simulink model "VDCHyd2022a"  (R2022a)
settings: Solver=daessc  StartTime=0.0  StopTime=simulationEndTime  FixedStep=0.001  RelTol=1e-2
values from neighbouring files (symbols this model uses):
  aux = thetaXrLB(i)    [initInertiaUpdate.m]
  Bc1_V = [0;0;0;0;0;0]    [InitializeSimulationParameters.m]
  Bc1_Vr = [0;0;0;0;0;0]    [InitializeSimulationParameters.m]
  D22Fr = [0;0;0;0;0;0]    [InitializeSimulationParameters.m]
  filtDF = init2ndOrderLowPassFilter(filtDF.cutOffFrequency,1,controller.dT)    [initializeLowPassFilters.m]
  filtDV = init2ndOrderLowPassFilter(filtDV.cutOffFrequency,1,controller.dT)    [initializeLowPassFilters.m]
  filtEnc = init2ndOrderLowPassFilter(filtEnc.cutOffFrequency,1,controller.dT)    [initializeLowPassFilters.m]
  filtPres = init2ndOrderLowPassFilter(filtPres.cutOffFrequency,1,controller.dT)    [initializeLowPassFilters.m]
  MODE = 1    [RUN_ME.m]
  s = tf('s')    [init2ndOrderLowPassFilter.m]
undefined symbols (not defined in the file or in its folder): B11_r_B11Tc1, B11_V, B11_Vr, B11Ftot_r, B12_r_B12Tc2, B12_Rot_Tc2, B12_U_Tc2, B12_V, B12_Vr, B12Ftot_r, B31_r_B31B41, B31_V, B31_Vr, B31FTot_r, B32_r_B32B42, B32_Rot_B42, B32_U_B42, B32_V, B32_Vr, B32FTot_r, B41_r_B41Tc1, B41_V, B41_Vr, B41FTot_r, B42_r_B42Tc2, B42_Rot_Tc2, B42_U_Tc2, B42_V, B42_Vr, B42FTot_r, B52_r_B52P32, B52_Rot_P32, B52_U_P32, B52_V, B52_Vr, B52Ftot_r, Bc1_r_Bc1B11, Bc1_r_Bc1B31, Bc1FTot_r, Bc2_r_Bc2B12, Bc2_r_Bc2B32, Bc2_Rot_B12, Bc2_Rot_B32, Bc2_U_B12, Bc2_U_B32, Bc2_V, Bc2_Vr, Bc2Tot_r, controller, cyl1, cyl2, cylT2, D22_V, D22_Vr, DiscIntNeverNeededParam, dq1, dq11, dq11r, dq12, dq12r ... (+119)
libraries: sm_lib x34, nesl_utility x15, simulink x11, dspinverses x1
(part 4 of 12)

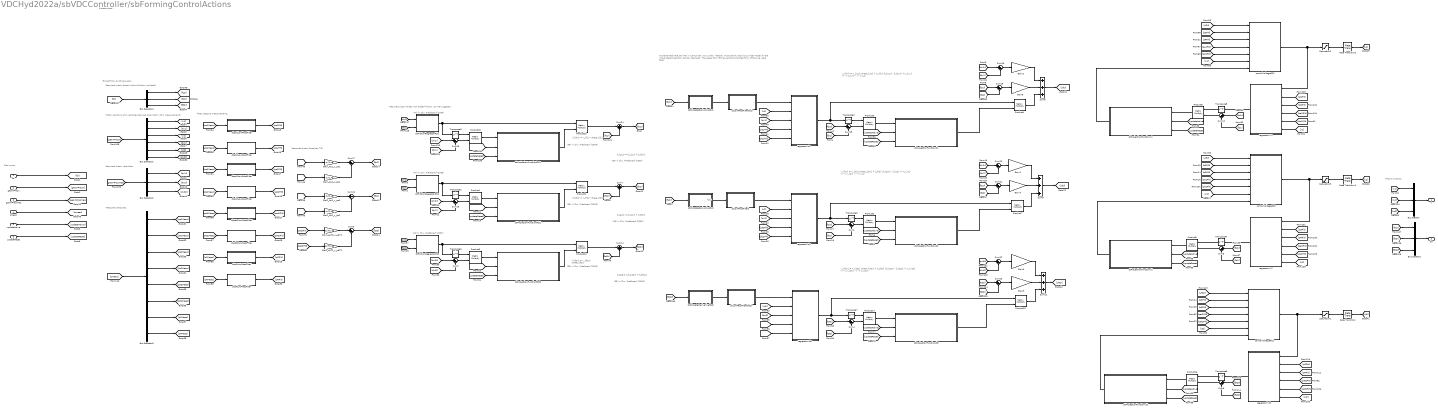
== system VDCHyd2022a/sbVDCController/sbFormingControlActions ==
  note: u_{f1r} = Y_{d1} \theta_{d1} + k_{f1} (f_{p1r} - f_{p1}) + k_{x1} (x^{'}_{1r} - x^{'}_1)
  note: fp2r
  note: Extract from existing buses...
  note: Get inputs...
  note: Pass to outputs...
  note: Process data...
  note: Filter pressure measurements.
  note: Measured piston force per (79).
  note: Required piston forces with added friction, as (78) suggests.
  note: Implemented here per (43) in (Lampinen, Koivumäki, Mattila): Improved Hydraulic Cylinder Model for the Virtual Decomposition Control Approach. The paper form (90) gives the simplified form of the one used here.
  note: Required piston forces (without friction included).
  note: Piston positions and velocities derived analytically from measurements.
  note: Required piston velocities.
  note: Measured pressures.
  note: f_{f1r} = Y_{f1}* \theta_{f1}
  note: f_{p1r} = f_{c1r} + f_{f1r}
  note: f_{f2r} = Y_{f2}* \theta_{f2}
  note: f_{p2r} = f_{c2r} + f_{f2r}
  note: f_{ft2r} = Y_{ft2}* \theta_{ft2}
  note: f_{pt2r} = f_{ct2r} + f_{ft2r}
  note: (40) in Zhu, Piedboeuf (2005)
  note: (40) in Zhu, Piedboeuf (2005)
  note: (40) in Zhu, Piedboeuf (2005)
  note: (39) in Zhu, Piedboeuf (2005)
  note: (39) in Zhu, Piedboeuf (2005)
  note: (39) in Zhu, Piedboeuf (2005)
  note: (38) in Zhu, Piedboeuf (2005)
  note: (38) in Zhu, Piedboeuf (2005)
  note: (38) in Zhu, Piedboeuf (2005)
  note: u_{f2r} = Y_{d2} \theta_{d2} + k_{f2} (f_{p2r} - f_{p2}) + k_{x2} (x^{'}_{2r} - x^{'}_2)
  note: u_{ft2r} = Y_{dt2} \theta_{dt2} + k_{ft2} (f_{pt2r} - f_{pt2}) + k_{xt2} (x^{'}_{t2r} - x^{'}_{t2})
  fcr : Inport
  geomPropX : Inport  Port=2
  geomPropXreq : Inport  Port=3
  pMeas : Inport  Port=4
  updateActive : Inport  Port=5
  updateReset : Inport  Port=6
  Bus Creator : BusCreator  Inputs=u1,u2,ut2
  Bus Creator1 : BusCreator  Inputs=fp1r,fp2r,fpt2r
  Bus Selector1 : BusSelector  OutputSignals=geomPropRS1.x1,geomPropRS1.dx1,geomPropRS2.x2,geomPropRS2.dx2,geomPropPS2.xt2,geomPropPS2.dxt2
  Bus Selector2 : BusSelector  OutputSignals=geomPropRS1req.dx1r,geomPropRS2req.dx2r,dxt2r
  Bus Selector3 : BusSelector  OutputSignals=pa1Measured,pb1Measured,pa2Measured,pb2Measured,pat2Measured,pbt2Measured,pSMeasured,pRMeasured
  Bus Selector4 : BusSelector  OutputSignals=fc1r,fc2r,fct2r
  Gain1 : Gain  Gain=controller.kx2
  Gain2 : Gain  Gain=controller.kx1
  Gain3 : Gain  Gain=controller.kxt2
  Gain4 : Gain  Gain=controller.kf2
  Gain8 : Gain  Gain=controller.kf1
  Gain9 : Gain  Gain=controller.kft2
  Gain_Aa1_x_pa1 : Gain  Gain=cyl1.Aa
  Gain_Aa2_x_pa2 : Gain  Gain=cyl2.Aa
  Gain_AaT2_x_paT2 : Gain  Gain=cylT2.Aa
  Gain_Ab1_x_pb1 : Gain  Gain=cyl1.Ab
  Gain_Ab2_x_pb2 : Gain  Gain=cyl2.Ab
  Gain_AbT2_x_pbT2 : Gain  Gain=cylT2.Ab
  Product{1..10,14..16,18,20} (15 alike) : Product  Multiplication=Matrix(*)
  Rate Transition : RateTransition  OutPortSampleTime=controller.dT
  Rate Transition1 : RateTransition  OutPortSampleTime=controller.dT
  Rate Transition2 : RateTransition  OutPortSampleTime=controller.dT
  Saturation1 : Saturate  UpperLimit=controller.ut2UppLim  LowerLimit=controller.ut2LowLim
  Saturation2 : Saturate  UpperLimit=controller.u1UppLim  LowerLimit=controller.u1LowLim
  Saturation3 : Saturate  UpperLimit=controller.u2UppLim  LowerLimit=controller.u2LowLim
  Sum{1..5,8,10,12..13,15..18,20..23,25} (18 alike) : Sum  Inputs=|+-
  Sum11 : Sum  Inputs=+++
  Sum14 : Sum  Inputs=|++
  Sum24 : Sum  Inputs=|++
  Sum6 : Sum  Inputs=+++
  Sum7 : Sum  Inputs=|++
  Sum9 : Sum  Inputs=+++
  Transpose{1..9} (9 alike) : Math  Operator=transpose
  controlVoltagePS2 : MATLAB Function  TreatAsAtomicUnit=on
  controlVoltageRS1 : MATLAB Function  TreatAsAtomicUnit=on
  controlVoltageRS2 : MATLAB Function  TreatAsAtomicUnit=on
  regressorYd1 : MATLAB Function  TreatAsAtomicUnit=on
  regressorYd2 : MATLAB Function  TreatAsAtomicUnit=on
  regressorYdt2 : MATLAB Function  TreatAsAtomicUnit=on
  regressorYv1 : MATLAB Function  TreatAsAtomicUnit=on
  regressorYv2 : MATLAB Function  TreatAsAtomicUnit=on
  regressorYvt2 : MATLAB Function  TreatAsAtomicUnit=on
  sbDiscreteDerivativefp1r : Subsystem
  sbDiscreteDerivativefp2r : Subsystem
  sbDiscreteDerivativefpt2r : Subsystem
  sbFrictionRegressorPS2 : Subsystem
  sbFrictionRegressorRS1 : Subsystem
  sbFrictionRegressorRS2 : Subsystem
  sbLowPassFilter2 : Subsystem
  sbLowPassFilterdfp1r : Subsystem
  sbLowPassFilterdfpt2r : Subsystem
  sbProjectionFunctiond1 : Subsystem
  sbProjectionFunctiond2 : Subsystem
  sbProjectionFunctiondt2 : Subsystem
  sbProjectionFunctionfRS1 : Subsystem
  sbProjectionFunctionfRS2 : Subsystem
  sbProjectionFunctionfRS3 : Subsystem
  sbProjectionFunctionv1 : Subsystem
  sbProjectionFunctionv2 : Subsystem
  sbProjectionFunctionvt2 : Subsystem
  sbpRLowPassFilter : Subsystem
  sbpSLowPassFilter : Subsystem
  sbpa1LowPassFilter : Subsystem
  sbpa2LowPassFilter : Subsystem
  sbpat2LowPassFilter : Subsystem
  sbpb1LowPassFilter : Subsystem
  sbpb2LowPassFilter : Subsystem
  sbpbt2LowPassFilter : Subsystem
  u : Outport
  fpr : Outport  Port=2
  wires:
  [uf1r] -> controlVoltageRS1/1(uf1r)  "uf1r"
  [fp2r] -> sbDiscreteDerivativefp2r/1(fp2r)  "fp2r"
  sbDiscreteDerivativefp2r/1(dfp2r) -> sbLowPassFilter2/1(dfp2r)  "dfp2r"
  sbDiscreteDerivativefp1r/1(dfp1r) -> sbLowPassFilterdfp1r/1(dfp1r)  "dfp1r"
  [fp1r] -> sbDiscreteDerivativefp1r/1(fp1r)  "fp1r"
  Sum20/1 -> Gain1/1
  Sum21/1 -> Gain4/1
  [fp2r] -> Sum21/1  "fp2r"
  [dx2] -> Sum20/2  "dx2"
  [dx2r] -> Sum20/1  "dx2r"
  [fp2] -> Sum21/2  "fp2"
  Gain1/1 -> Sum9/1
  Gain4/1 -> Sum9/2
  Product7/1 -> Sum9/3
  sbLowPassFilter2/1(dfp2rFilt) -> regressorYd2/1(dfp2r)  "dfp2rFilt"
  [x2] -> regressorYd2/2(x2)  "x2"
  [dx2] -> regressorYd2/3(dx2)  "dx2"
  [pa2Filt] -> regressorYd2/4(pa2)  "pa2"
  [pb2Filt] -> regressorYd2/5(pb2)  "pb2"
  regressorYd2/1(Yd2) -> Product7/1, Transpose3/1  "Yd2"
  [fp2r] -> Sum1/1  "fp2r"
  Transpose3/1 -> Product6/1
  Sum1/1 -> Product6/2
  Product6/1 -> sbProjectionFunctiond2/1(sd2)  "sd2"
  [fp2] -> Sum1/2  "fp2"
  sbProjectionFunctiond2/1(thetad2) -> Product7/2  "thetad2"
  Gain8/1 -> Sum6/2
  Gain2/1 -> Sum6/1
  [fp1] -> Sum18/2  "fp1"
  [dx1r] -> Sum16/1  "dx1r"
  [dx1] -> Sum16/2  "dx1"
  sbProjectionFunctiond1/1(thetad1) -> Product4/2  "thetad1"
  [updateReset] -> sbProjectionFunctiond1/3(updateReset)  "updateReset"
  [updateActive] -> sbProjectionFunctiond1/2(updateActive)  "updateActive"
  updateReset/1 -> [updateReset]  "updateReset"
  updateActive/1 -> [updateActive]  "updateActive"
  [fp1] -> Sum15/2  "fp1"
  Gain_Aa1_x_pa1/1 -> Sum17/1
  [pb1Filt] -> Gain_Ab1_x_pb1/1  "pb1Filt"
  Gain_Ab1_x_pb1/1 -> Sum17/2
  [pa1Filt] -> Gain_Aa1_x_pa1/1  "pa1Filt"
  [pa2Filt] -> Gain_Aa2_x_pa2/1  "pa2Filt"
  Gain_Ab2_x_pb2/1 -> Sum10/2
  [pb2Filt] -> Gain_Ab2_x_pb2/1  "pb2Filt"
  Gain_Aa2_x_pa2/1 -> Sum10/1
  sbpa1LowPassFilter/1(pa1Filt) -> [pa1Filt]  "pa1Filt"
  sbpb1LowPassFilter/1(pb1Filt) -> [pb1Filt]  "pb1Filt"
  sbpa2LowPassFilter/1(pa2Filt) -> [pa2Filt]  "pa2Filt"
  sbpb2LowPassFilter/1(pb2Filt) -> [pb2Filt]  "pb2Filt"
  sbpSLowPassFilter/1(pSFilt) -> [pSFilt]  "pSFilt"
  [pSMeas] -> sbpSLowPassFilter/1(pSMeas)  "pSMeas"
  [pb2Meas] -> sbpb2LowPassFilter/1(pb2Meas)  "pb2Meas"
  [pa2Meas] -> sbpa2LowPassFilter/1(pa2Meas)  "pa2Meas"
  [pb1Meas] -> sbpb1LowPassFilter/1(pb1Meas)  "pb1Meas"
  [pa1Meas] -> sbpa1LowPassFilter/1(pa1Meas)  "pa1Meas"
  sbProjectionFunctionv1/1(thetav1) -> controlVoltageRS1/7(thetav1)  "thetav1"
  [fp1r] -> Sum18/1  "fp1r"
  Sum18/1 -> Gain8/1
  Sum16/1 -> Gain2/1
  Product3/1 -> sbProjectionFunctiond1/1(sd1)  "sd1"
  Sum15/1 -> Product3/2
  Transpose2/1 -> Product3/1
  [fp1r] -> Sum15/1  "fp1r"
  regressorYd1/1(Yd1) -> Transpose2/1, Product4/1  "Yd1"
  [pb1Filt] -> regressorYd1/5(pb1)  "pb1Filt"
  [pa1Filt] -> regressorYd1/4(pa1)  "pa1Filt"
  [dx1] -> regressorYd1/3(dx1)  "dx1"
  [x1] -> regressorYd1/2(x1)  "x1"
  sbLowPassFilterdfp1r/1(dfp1rFilt) -> regressorYd1/1(dfp1r)  "dfp1r"
  controlVoltageRS1/1(u1) -> Saturation2/1, regressorYv1/1(u1)  "u1"
  [pSFilt] -> controlVoltageRS1/2(pS)  "pSFilt"
  [x1] -> controlVoltageRS1/6(x1)  "x1"
  [pb1Filt] -> controlVoltageRS1/5(pb1)  "pb1Filt"
  [pa1Filt] -> controlVoltageRS1/4(pa1)  "pa1Filt"
  [pb1Filt] -> regressorYv1/5(pb1)  "pb1Filt"
  [x1] -> regressorYv1/6(x1)  "x1"
  [pSFilt] -> regressorYv1/2(pS)  "pSFilt"
  [pa1Filt] -> regressorYv1/4(pa1)  "pa1Filt"
  Product9/1 -> sbProjectionFunctionv1/1(sv1)  "sv1"
  Transpose5/1 -> Product9/1
  [fp1] -> Sum12/2  "fp1"
  Sum12/1 -> Product9/2
  [fp1r] -> Sum12/1  "fp1r"
  regressorYv1/1(Yv1) -> Transpose5/1  "Yv1"
  Sum17/1 -> [fp1]  "fp1"
  Sum10/1 -> [fp2]  "fp2"
  Sum6/1 -> [uf1r]  "uf1r"
  Sum9/1 -> [uf2r]  "uf2r"
  Product4/1 -> Sum6/3
  Sum3/1 -> [fpt2]  "fpt2"
  Gain_AaT2_x_paT2/1 -> Sum3/1
  [pbt2Filt] -> Gain_AbT2_x_pbT2/1
  Gain_AbT2_x_pbT2/1 -> Sum3/2
  [pat2Filt] -> Gain_AaT2_x_paT2/1
  [u2] -> Bus Creator/2  "u2"
  [u1] -> Bus Creator/1  "u1"
  [ut2] -> Bus Creator/3  "ut2"
  Bus Creator/1 -> u/1  "u"
  [pat2Meas] -> sbpat2LowPassFilter/1(pat2Meas)  "pat2Meas"
  [pbt2Meas] -> sbpbt2LowPassFilter/1(pbt2Meas)  "pbt2Meas"
  sbpbt2LowPassFilter/1(pbt2Filt) -> [pbt2Filt]  "pbt2Filt"
  sbpat2LowPassFilter/1(pat2Filt) -> [pat2Filt]  "pat2Filt"
  [pRMeas] -> sbpRLowPassFilter/1(pRMeas)  "pRMeas"
  sbpRLowPassFilter/1(pRFilt) -> [pRFilt]  "pRFilt"
  sbProjectionFunctiondt2/1(thetadT2) -> Product15/2
  [fpt2] -> Sum4/2  "fpt2"
  Product14/1 -> sbProjectionFunctiondt2/1(sdt2)  "sdt2"
  Sum4/1 -> Product14/2
  Transpose7/1 -> Product14/1
  [fpt2r] -> Sum4/1  "fpt2r"
  regressorYdt2/1(Ydt2) -> Transpose7/1, Product15/1  "Ydt2"
  [pbt2Filt] -> regressorYdt2/5(pbt2)  "pbt2Filt"
  [pat2Filt] -> regressorYdt2/4(pat2)  "pat2Filt"
  [dxt2] -> regressorYdt2/3(dxt2)  "dxt2"
  [xt2] -> regressorYdt2/2(xt2)  "xt2"
  sbLowPassFilterdfpt2r/1(dfpt2rFilt) -> regressorYdt2/1(dfpt2r)  "dfpt2rFilt"
  sbDiscreteDerivativefpt2r/1(dfpt2r) -> sbLowPassFilterdfpt2r/1(dfpt2r)  "dfpt2r"
  [fpt2r] -> sbDiscreteDerivativefpt2r/1(fpt2r)  "fpt2r"
  [pRFilt] -> controlVoltageRS1/3(pR)  "pRFilt"
  [pRFilt] -> regressorYv1/3(pR)  "pRFilt"
  [pRFilt] -> controlVoltageRS2/3(pR)  "pRFilt"
  [x2] -> controlVoltageRS2/6(x2)  "x2"
  [pSFilt] -> controlVoltageRS2/2(pS)  "pSFilt"
  [x2] -> regressorYv2/6(x2)  "x2"
  [fp2r] -> Sum5/1  "fp2r"
  [pa2Filt] -> controlVoltageRS2/4(pa2)  "pa2Filt"
  controlVoltageRS2/1(u2) -> Saturation3/1, regressorYv2/1(u2)  "u2"
  [pRFilt] -> regressorYv2/3(pR)  "pRFilt"
  [pb2Filt] -> regressorYv2/5(pb2)  "pb2Filt"
  Sum5/1 -> Product8/2
  regressorYv2/1(Yv2) -> Transpose4/1  "Yv2"
  [fp2] -> Sum5/2  "fp2"
  Transpose4/1 -> Product8/1
  [pSFilt] -> regressorYv2/2(pS)  "pSFilt"
  [pb2Filt] -> controlVoltageRS2/5(pb2)  "pb2Filt"
  [pa2Filt] -> regressorYv2/4(pa2)  "pa2Filt"
  sbProjectionFunctionv2/1(thetav2) -> controlVoltageRS2/7(thetav2)  "thetav2"
  Product8/1 -> sbProjectionFunctionv2/1(sv2)  "sv2"
  [uf2r] -> controlVoltageRS2/1(uf2r)  "uf2r"
  [uft2r] -> controlVoltagePS2/1(uft2r)  "uft2r"
  Product16/1 -> sbProjectionFunctionvt2/1(svt2)  "svt2"
  sbProjectionFunctionvt2/1(thetavt2) -> controlVoltagePS2/7(thetavt2)  "thetavt2"
  [pat2Filt] -> regressorYvt2/4(pat2)  "pat2Filt"
  [pbt2Filt] -> controlVoltagePS2/5(pbt2)  "pbt2Filt"
  [pSFilt] -> regressorYvt2/2(pS)  "pSFilt"
  Transpose8/1 -> Product16/1
  [fpt2] -> Sum8/2  "fpt2"
  regressorYvt2/1(Yvt2) -> Transpose8/1  "Yvt2"
  Sum8/1 -> Product16/2
  [pbt2Filt] -> regressorYvt2/5(pbt2)  "pbt2Filt"
  [pRFilt] -> regressorYvt2/3(pR)  "pRFilt"
  controlVoltagePS2/1(ut2) -> regressorYvt2/1(ut2), Saturation1/1  "ut2"
  [pat2Filt] -> controlVoltagePS2/4(pat2)  "pat2Filt"
  [fpt2r] -> Sum8/1  "fpt2r"
  [xt2] -> regressorYvt2/6(xt2)  "xt2"
  [pSFilt] -> controlVoltagePS2/2(pS)  "pSFilt"
  [xt2] -> controlVoltagePS2/6(xt2)  "xt2"
  [pRFilt] -> controlVoltagePS2/3(pR)  "pRFilt"
  Sum11/1 -> [uft2r]
  Product15/1 -> Sum11/3
  Gain9/1 -> Sum11/2
  Gain3/1 -> Sum11/1
  [fpt2] -> Sum23/2  "fpt2"
  [dxt2r] -> Sum22/1  "dxt2r"
  [dxt2] -> Sum22/2  "dxt2"
  [fpt2r] -> Sum23/1  "fpt2r"
  Sum23/1 -> Gain9/1
  Sum22/1 -> Gain3/1
  [fp2r] -> Bus Creator1/2  "fp2r"
  [fp1r] -> Bus Creator1/1  "fp1r"
  [fpt2r] -> Bus Creator1/3  "fpt2r"
  Bus Creator1/1 -> fpr/1  "fpr"
  Rate Transition/1 -> [ut2]  "ut2"
  Rate Transition1/1 -> [u2]  "u2"
  Rate Transition2/1 -> [u1]
  Saturation1/1 -> Rate Transition/1  "ut2"
  Saturation3/1 -> Rate Transition1/1  "u2"
  Saturation2/1 -> Rate Transition2/1  "u1"
  Bus Selector4/3 -> [fct2r]  "<fct2r>"
  [fcr] -> Bus Selector4/1  "fcr"
  Bus Selector4/1 -> [fc1r]  "<fc1r>"
  Bus Selector4/2 -> [fc2r]  "<fc2r>"
  fcr/1 -> [fcr]  "fcr"
  Bus Selector1/4 -> [dx2]  "<dx2>"
  Bus Selector1/2 -> [dx1]  "<dx1>"
  Bus Selector1/3 -> [x2]  "<x2>"
  Bus Selector1/5 -> [xt2]  "<xt2>"
  Bus Selector1/6 -> [dxt2]  "<dxt2>"
  Bus Selector1/1 -> [x1]  "<x1>"
  [geomPropX] -> Bus Selector1/1  "geomPropX"
  geomPropX/1 -> [geomPropX]  "geomPropX"
  Bus Selector2/1 -> [dx1r]  "<dx1r>"
  [geomPropXreq] -> Bus Selector2/1  "geomPropXreq"
  Bus Selector2/2 -> [dx2r]  "<dx2r>"
  Bus Selector2/3 -> [dxt2r]  "<dxt2r>"
  geomPropXreq/1 -> [geomPropXreq]  "geomPropXreq"
  Bus Selector3/6 -> [pbt2Meas]  "<pbt2Measured>"
  Bus Selector3/3 -> [pa2Meas]  "<pa2Measured>"
  [pmeas] -> Bus Selector3/1  "pMeas"
  Bus Selector3/8 -> [pRMeas]  "<pRMeasured>"
  Bus Selector3/4 -> [pb2Meas]  "<pb2Measured>"
  Bus Selector3/7 -> [pSMeas]  "<pSMeasured>"
  Bus Selector3/1 -> [pa1Meas]  "<pa1Measured>"
  Bus Selector3/5 -> [pat2Meas]  "<pat2Measured>"
  Bus Selector3/2 -> [pb1Meas]  "<pb1Measured>"
  pMeas/1 -> [pmeas]  "pMeas"
  [updateReset] -> sbProjectionFunctiond2/3(updateReset)  "updateReset"
  [updateActive] -> sbProjectionFunctiond2/2(updateActive)  "updateActive"
  [updateActive] -> sbProjectionFunctiondt2/2(updateActive)  "updateActive"
  [updateReset] -> sbProjectionFunctiondt2/3(updateReset)  "updateReset"
  [updateReset] -> sbProjectionFunctionv1/3(updateReset)  "updateReset"
  [updateActive] -> sbProjectionFunctionv1/2(updateActive)  "updateActive"
  [updateReset] -> sbProjectionFunctionv2/3(updateReset)  "updateReset"
  [updateActive] -> sbProjectionFunctionv2/2(updateActive)  "updateActive"
  [updateActive] -> sbProjectionFunctionvt2/2(updateActive)  "updateActive"
  [updateReset] -> sbProjectionFunctionvt2/3(updateReset)  "updateReset"
  [dx1] -> sbFrictionRegressorRS1/1(dx1)  "dx1"
  [fp1] -> sbFrictionRegressorRS1/2(fp1)  "fp1"
  Product20/1 -> Sum24/1  "ff1r"
  Sum25/1 -> Product18/2
  Product18/1 -> sbProjectionFunctionfRS1/1(sf1)  "sf1"
  Transpose9/1 -> Product18/1
  [dx1] -> Sum25/2  "dx1"
  [fc1r] -> Sum24/2  "fc1r"
  [dx1r] -> Sum25/1  "dx1r"
  sbFrictionRegressorRS1/1(Yf1) -> Transpose9/1, Product20/1  "Yf1"
  sbProjectionFunctionfRS1/1(thetaf1) -> Product20/2  "thetaf1"
  Sum24/1 -> [fp1r]  "fp1r"
  [updateActive] -> sbProjectionFunctionfRS1/2(updateActive)  "updateActive"
  [updateReset] -> sbProjectionFunctionfRS1/3(updateReset)  "updateReset"
  [updateReset] -> sbProjectionFunctionfRS2/3(updateReset)  "updateReset"
  [updateActive] -> sbProjectionFunctionfRS2/2(updateActive)  "updateActive"
  Sum7/1 -> [fp2r]  "fp2r"
  sbProjectionFunctionfRS2/1(thetaf2) -> Product2/2  "thetaf2"
  sbFrictionRegressorRS2/1(Yf2) -> Product2/1, Transpose1/1  "Yf2"
  [dx2r] -> Sum13/1  "dx2r"
  [fc2r] -> Sum7/2  "fc2r"
  [dx2] -> Sum13/2  "dx2"
  Transpose1/1 -> Product1/1
  Product1/1 -> sbProjectionFunctionfRS2/1(sf2)  "sf2"
  Sum13/1 -> Product1/2
  Product2/1 -> Sum7/1  "ff2r"
  [fp2] -> sbFrictionRegressorRS2/2(fp2)  "fp2"
  [dx2] -> sbFrictionRegressorRS2/1(dx2)  "dx2"
  [dxt2] -> sbFrictionRegressorPS2/1(dxt2)  "dxt2"
  [fpt2] -> sbFrictionRegressorPS2/2(fpt2)  "fpt2"
  Product10/1 -> Sum14/1  "fft2r"
  Sum2/1 -> Product5/2
  Product5/1 -> sbProjectionFunctionfRS3/1(sfT2)  "sfT2"
  Transpose6/1 -> Product5/1
  [dxt2] -> Sum2/2  "dxt2"
  [fct2r] -> Sum14/2  "fct2r"
  [dxt2r] -> Sum2/1  "dxt2r"
  sbFrictionRegressorPS2/1(Yft2) -> Transpose6/1, Product10/1  "YfT2"
  sbProjectionFunctionfRS3/1(thetafT2) -> Product10/2  "thetafT2"
  Sum14/1 -> [fpt2r]  "fpt2r"
  [updateActive] -> sbProjectionFunctionfRS3/2(updateActive)  "updateActive"
  [updateReset] -> sbProjectionFunctionfRS3/3(updateReset)  "updateReset"

== system VDCHyd2022a/sbVDCController/sbForwardKinematics ==
  note: Get inputs...
  note: Calculate the end-effector position in the world {W} frame...
  note: Select from existing buses...
  note: Process data...
  note: Pass to outputs...
  PosVecs_Sx : Inport
  WRotX : Inport  Port=2
  Bus Selector : BusSelector  OutputSignals=posVecsRS1.W_r_WBc1,posVecsRS1.Bc1_r_Bc1B11,posVecsRS1.B11_r_B11Tc1,posVecsRS1.Tc1_r_Tc1Bc2,posVecsRS2.Bc2_r_Bc2B12,posVecsRS2.B12_r_B12Tc2,posVecsRS2.Tc2_r_Tc2P22,posVecsPS2.P22_r_P22B52,posVecsPS2.B52_r_B52P32,posVecsPS2.P32_r_P32D22
  Bus Selector1 : BusSelector  OutputSignals=WRotXRS1.W_Rot_Bc1,WRotXRS1.W_Rot_B11,WRotXRS1.W_Rot_Tc1,WRotXRS1.W_Rot_Bc2,WRotXRS2.W_Rot_B12,WRotXRS2.W_Rot_Tc2,WRotXRS2.W_Rot_P22,WRotXPS2.W_Rot_B52,WRotXPS2.W_Rot_P32
  Product{2..10} (9 alike) : Product  Multiplication=Matrix(*)
  Sum : Sum  Inputs=|++++++++++
  WrWD22 : Outport
  wires:
  Product10/1 -> Sum/10
  Product9/1 -> Sum/9
  Product8/1 -> Sum/8
  Product7/1 -> Sum/7
  Product6/1 -> Sum/6
  Product5/1 -> Sum/5
  Product4/1 -> Sum/4
  Product3/1 -> Sum/3
  Product2/1 -> Sum/2
  [rWBc1] -> Sum/1
  Bus Selector/1 -> [rWBc1]  "<W_r_WBc1>"
  [WRotP32] -> Product10/1
  [rP32G] -> Product10/2
  Bus Selector/10 -> [rP32G]  "<P32_r_P32D22>"
  Bus Selector1/9 -> [WRotP32]  "<W_Rot_P32>"
  [rB52P32] -> Product9/2
  [WRotB52] -> Product9/1
  [WRotP22] -> Product8/1
  [rP22B52] -> Product8/2
  Bus Selector/9 -> [rB52P32]  "<B52_r_B52P32>"
  Bus Selector/8 -> [rP22B52]  "<P22_r_P22B52>"
  Bus Selector1/8 -> [WRotB52]  "<W_Rot_B52>"
  Bus Selector1/7 -> [WRotP22]  "<W_Rot_P22>"
  [WrWD22] -> WrWD22/1  "WrWD22"
  Sum/1 -> [WrWD22]  "WrWD22"
  [WRotBc1] -> Product2/1
  [WRotB11] -> Product3/1
  [WRotTc1] -> Product4/1
  [WRotBc2] -> Product5/1
  [WRotB12] -> Product6/1
  [WRotTc2] -> Product7/1
  Bus Selector1/6 -> [WRotTc2]  "<W_Rot_Tc2>"
  Bus Selector1/5 -> [WRotB12]  "<W_Rot_B12>"
  Bus Selector1/4 -> [WRotBc2]  "<W_Rot_Bc2>"
  Bus Selector1/3 -> [WRotTc1]  "<W_Rot_Tc1>"
  Bus Selector1/2 -> [WRotB11]  "<W_Rot_B11>"
  Bus Selector1/1 -> [WRotBc1]  "<W_Rot_Bc1>"
  [WRotXSx] -> Bus Selector1/1  "WRotX_Sx"
  [rTc2P22] -> Product7/2
  [rB12Tc2] -> Product6/2
  [rBc2B12] -> Product5/2
  [rTc1Bc2] -> Product4/2
  [rB11Tc1] -> Product3/2
  [rBc1B11] -> Product2/2
  Bus Selector/4 -> [rTc1Bc2]  "<Tc1_r_Tc1Bc2>"
  Bus Selector/5 -> [rBc2B12]  "<Bc2_r_Bc2B12>"
  Bus Selector/6 -> [rB12Tc2]  "<B12_r_B12Tc2>"
  Bus Selector/7 -> [rTc2P22]  "<Tc2_r_Tc2P22>"
  Bus Selector/3 -> [rB11Tc1]  "<B11_r_B11Tc1>"
  Bus Selector/2 -> [rBc1B11]  "<Bc1_r_Bc1B11>"
  [PosVecsSx] -> Bus Selector/1  "PosVecs_Sx"
  PosVecs_Sx/1 -> [PosVecsSx]  "PosVecs_Sx"
  WRotX/1 -> [WRotXSx]  "WRot_Sx"

== system VDCHyd2022a/sbHydraulicElements/sbHosesAndActuatorPS2/sbChamberAPressure ==
  Qa : Inport
  Ql : Inport  Port=2
  xp : Inport  Port=3
  dxp : Inport  Port=4
  Constant4 : Constant  Value=hosingT2.V0a
  Divide : Product  Inputs=*/
  Gain : Gain  Gain=oil.B
  Gain1 : Gain  Gain=cylT2.Aa
  Gain2 : Gain  Gain=cylT2.Aa
  Integrator : Integrator  InitialCondition=initVals.pat20  LimitOutput=on  UpperSaturationLimit=pres.supply  LowerSaturationLimit=pres.return
  Sum : Sum  Inputs=|+--
  Sum1 : Sum  Inputs=|++
  pa : Outport
  wires:
  Gain2/1 -> Sum/2
  Qa/1 -> Sum/1  "Qa"
  Integrator/1 -> pa/1  "pa"
  Sum/1 -> Gain/1
  Constant4/1 -> Sum1/1
  xp/1 -> Gain1/1  "xp"
  Divide/1 -> Integrator/1  "dpa"
  Gain1/1 -> Sum1/2
  Gain/1 -> Divide/1
  Sum1/1 -> Divide/2
  Ql/1 -> Sum/3  "Ql"
  dxp/1 -> Gain2/1  "dxp"

== system VDCHyd2022a/sbHydraulicElements/sbHosesAndActuatorPS2/sbChamberBPressure ==
  Qb : Inport
  Ql : Inport  Port=2
  xp : Inport  Port=3
  dxp : Inport  Port=4
  Constant : Constant  Value=cylT2.sp
  Constant4 : Constant  Value=hosingT2.V0b
  Divide : Product  Inputs=*/
  Gain : Gain  Gain=oil.B
  Gain1 : Gain  Gain=cylT2.Ab
  Gain2 : Gain  Gain=cylT2.Ab
  Integrator : Integrator  InitialCondition=initVals.pbt20  LimitOutput=on  UpperSaturationLimit=pres.supply  LowerSaturationLimit=pres.return
  Sum : Sum  Inputs=|+++
  Sum1 : Sum  Inputs=|++
  Sum2 : Sum  Inputs=|-+
  pb : Outport
  wires:
  Constant/1 -> Sum2/2
  Sum2/1 -> Gain1/1
  xp/1 -> Sum2/1  "xp"
  Ql/1 -> Sum/3  "Ql"
  Sum1/1 -> Divide/2
  Gain/1 -> Divide/1
  Gain1/1 -> Sum1/2
  Divide/1 -> Integrator/1  "dpb"
  Constant4/1 -> Sum1/1
  Sum/1 -> Gain/1
  Integrator/1 -> pb/1  "pb"
  Qb/1 -> Sum/1  "Qb"
  Gain2/1 -> Sum/2
  dxp/1 -> Gain2/1  "dxp"

== system VDCHyd2022a/sbHydraulicElements/sbHosesAndActuatorPS2/sbLeakageFlow ==
  pa : Inport
  pb : Inport  Port=2
  Gain2 : Gain  Gain=cylT2.cl
  Sum4 : Sum  Inputs=|+-
  Ql : Outport
  wires:
  Sum4/1 -> Gain2/1
  Gain2/1 -> Ql/1  "Ql"
  pb/1 -> Sum4/2  "pb"
  pa/1 -> Sum4/1  "pa"

== system VDCHyd2022a/sbHydraulicElements/sbHosesAndActuatorRS1/sbChamberAPressure ==
  Qa : Inport
  Ql : Inport  Port=2
  xp : Inport  Port=3
  dxp : Inport  Port=4
  Constant4 : Constant  Value=hosing1.V0a
  Divide : Product  Inputs=*/
  Gain : Gain  Gain=oil.B
  Gain1 : Gain  Gain=cyl1.Aa
  Gain2 : Gain  Gain=cyl1.Aa
  Integrator : Integrator  InitialCondition=initVals.pa10  LimitOutput=on  UpperSaturationLimit=pres.supply  LowerSaturationLimit=pres.return
  Sum : Sum  Inputs=|+--
  Sum1 : Sum  Inputs=|++
  pa : Outport
  wires:
  Gain2/1 -> Sum/2
  Qa/1 -> Sum/1  "Qa"
  Integrator/1 -> pa/1  "pa"
  Sum/1 -> Gain/1
  Constant4/1 -> Sum1/1
  xp/1 -> Gain1/1  "xp"
  Divide/1 -> Integrator/1  "dpa"
  Gain1/1 -> Sum1/2
  Gain/1 -> Divide/1
  Sum1/1 -> Divide/2
  Ql/1 -> Sum/3  "Ql"
  dxp/1 -> Gain2/1  "dxp"

== system VDCHyd2022a/sbHydraulicElements/sbHosesAndActuatorRS1/sbChamberBPressure ==
  Qb : Inport
  Ql : Inport  Port=2
  xp : Inport  Port=3
  dxp : Inport  Port=4
  Constant : Constant  Value=cyl1.sp
  Constant4 : Constant  Value=hosing1.V0b
  Divide : Product  Inputs=*/
  Gain : Gain  Gain=oil.B
  Gain1 : Gain  Gain=cyl1.Ab
  Gain2 : Gain  Gain=cyl1.Ab
  Integrator : Integrator  InitialCondition=initVals.pb10  LimitOutput=on  UpperSaturationLimit=pres.supply  LowerSaturationLimit=pres.return
  Sum : Sum  Inputs=|+++
  Sum1 : Sum  Inputs=|++
  Sum2 : Sum  Inputs=|-+
  pb : Outport
  wires:
  Constant/1 -> Sum2/2
  Sum2/1 -> Gain1/1
  xp/1 -> Sum2/1  "xp"
  dxp/1 -> Gain2/1  "dxp"
  Ql/1 -> Sum/3  "Ql"
  Sum1/1 -> Divide/2
  Gain/1 -> Divide/1
  Divide/1 -> Integrator/1  "dpb"
  Constant4/1 -> Sum1/1
  Sum/1 -> Gain/1
  Integrator/1 -> pb/1  "pb"
  Qb/1 -> Sum/1  "Qb"
  Gain2/1 -> Sum/2
  Gain1/1 -> Sum1/2

== system VDCHyd2022a/sbHydraulicElements/sbHosesAndActuatorRS1/sbLeakageFlow ==
  pa : Inport
  pb : Inport  Port=2
  Gain2 : Gain  Gain=cyl1.cl
  Sum4 : Sum  Inputs=|+-
  Ql : Outport
  wires:
  Sum4/1 -> Gain2/1
  Gain2/1 -> Ql/1  "Ql"
  pb/1 -> Sum4/2  "pb"
  pa/1 -> Sum4/1  "pa"

== system VDCHyd2022a/sbHydraulicElements/sbHosesAndActuatorRS2/sbChamberAPressure ==
  Qa : Inport
  Ql : Inport  Port=2
  xp : Inport  Port=3
  dxp : Inport  Port=4
  Constant4 : Constant  Value=hosing2.V0a
  Divide : Product  Inputs=*/
  Gain : Gain  Gain=oil.B
  Gain1 : Gain  Gain=cyl2.Aa
  Gain2 : Gain  Gain=cyl2.Aa
  Integrator : Integrator  InitialCondition=initVals.pa20  LimitOutput=on  UpperSaturationLimit=pres.supply  LowerSaturationLimit=pres.return
  Sum : Sum  Inputs=|+--
  Sum1 : Sum  Inputs=|++
  pa : Outport
  wires:
  dxp/1 -> Gain2/1  "dxp"
  Ql/1 -> Sum/3  "Ql"
  Sum1/1 -> Divide/2
  Gain/1 -> Divide/1
  Gain1/1 -> Sum1/2
  Divide/1 -> Integrator/1  "dpa"
  xp/1 -> Gain1/1  "xp"
  Constant4/1 -> Sum1/1
  Sum/1 -> Gain/1
  Integrator/1 -> pa/1  "pa"
  Qa/1 -> Sum/1  "Qa"
  Gain2/1 -> Sum/2

== system VDCHyd2022a/sbHydraulicElements/sbHosesAndActuatorRS2/sbChamberBPressure ==
  Qb : Inport
  Ql : Inport  Port=2
  xp : Inport  Port=3
  dxp : Inport  Port=4
  Constant : Constant  Value=cyl2.sp
  Constant4 : Constant  Value=hosing2.V0b
  Divide : Product  Inputs=*/
  Gain : Gain  Gain=oil.B
  Gain1 : Gain  Gain=cyl2.Ab
  Gain2 : Gain  Gain=cyl2.Ab
  Integrator : Integrator  InitialCondition=initVals.pb20  LimitOutput=on  UpperSaturationLimit=pres.supply  LowerSaturationLimit=pres.return
  Sum : Sum  Inputs=|+++
  Sum1 : Sum  Inputs=|++
  Sum2 : Sum  Inputs=|-+
  pb : Outport
  wires:
  Gain2/1 -> Sum/2
  Qb/1 -> Sum/1  "Qb"
  Integrator/1 -> pb/1  "pb"
  Sum/1 -> Gain/1
  Constant4/1 -> Sum1/1
  Divide/1 -> Integrator/1  "dpb"
  Gain1/1 -> Sum1/2
  Gain/1 -> Divide/1
  Sum1/1 -> Divide/2
  Ql/1 -> Sum/3  "Ql"
  dxp/1 -> Gain2/1  "dxp"
  xp/1 -> Sum2/1  "xp"
  Sum2/1 -> Gain1/1
  Constant/1 -> Sum2/2

== system VDCHyd2022a/sbHydraulicElements/sbHosesAndActuatorRS2/sbLeakageFlow ==
  pa : Inport
  pb : Inport  Port=2
  Gain2 : Gain  Gain=cyl2.cl
  Sum4 : Sum  Inputs=|+-
  Ql : Outport
  wires:
  pa/1 -> Sum4/1  "pa"
  pb/1 -> Sum4/2  "pb"
  Gain2/1 -> Ql/1  "Ql"
  Sum4/1 -> Gain2/1

== system VDCHyd2022a/sbHydraulicManipulatorSimscape/sbLiftCylinderAndLiftPiston/sbFrictionForceRS1 ==
  note: (41) in Zhu, Piedboeuf (2005)
  note: (40) in Zhu, Piedboeuf (2005)
  dx1 : Inport
  fp1 : Inport  Port=2
  Constant1 : Constant  Value=update.thetaf1Nominal
  Product10 : Product  Multiplication=Matrix(*)
  sbFrictionRegressorRS1 : Subsystem
  ff1 : Outport
  wires:
  dx1/1 -> sbFrictionRegressorRS1/1(dx1)  "dx1"
  fp1/1 -> sbFrictionRegressorRS1/2(fp1)  "fp1"
  sbFrictionRegressorRS1/1(Yf1) -> Product10/1  "Yf1"
  Constant1/1 -> Product10/2  "thetaf1Nominal"
  Product10/1 -> ff1/1  "ff1"

== system VDCHyd2022a/sbHydraulicManipulatorSimscape/sbPrismaticJointCylinderAndPiston/sbFrictionForcePS2 ==
  note: (41) in Zhu, Piedboeuf (2005)
  note: (40) in Zhu, Piedboeuf (2005)
  dx2t : Inport
  fpt2 : Inport  Port=2
  Constant1 : Constant  Value=update.thetafT2Nominal
  Product10 : Product  Multiplication=Matrix(*)
  sbFrictionRegressorPS2 : Subsystem
  fft2 : Outport
  wires:
  dx2t/1 -> sbFrictionRegressorPS2/1(dxt2)  "dxt2"
  fpt2/1 -> sbFrictionRegressorPS2/2(fpt2)  "fpt2"
  sbFrictionRegressorPS2/1(Yft2) -> Product10/1  "Yft2"
  Constant1/1 -> Product10/2  "thetafT2Nominal"
  Product10/1 -> fft2/1  "fft2"

== system VDCHyd2022a/sbHydraulicManipulatorSimscape/sbTiltCylinderAndTiltPiston/sbFrictionForceRS2 ==
  note: (41) in Zhu, Piedboeuf (2005)
  note: (40) in Zhu, Piedboeuf (2005)
  dx2 : Inport
  fp2 : Inport  Port=2
  Constant1 : Constant  Value=update.thetaf2Nominal
  Product10 : Product  Multiplication=Matrix(*)
  sbFrictionRegressorRS2 : Subsystem
  ff2 : Outport
  wires:
  dx2/1 -> sbFrictionRegressorRS2/1(dx2)  "dx2"
  fp2/1 -> sbFrictionRegressorRS2/2(fp2)  "fp2"
  sbFrictionRegressorRS2/1(Yf2) -> Product10/1  "Yf2"
  Constant1/1 -> Product10/2  "thetaf2Nominal"
  Product10/1 -> ff2/1  "ff2"

== system VDCHyd2022a/sbVDCController/sbFormAnalyticQuantities/sbPrismaticSegment2 ==
  note: Process data...
  note: Get inputs...
  note: Pass to outputs...
  note: POSITION VECTORS
  note: Calculate kinematic quantities (18) - (23) in the prismatic segment 2 (PS2).
  note: Form relevant velocity/force transformation matrices...
  note: Form relevant rotation matrices...
  note: Form relevant required linear/angular velocities per (47) - (48).
  note: Form relevant position vectors...
  note: VELOCITY/FORCE TRANSFORMATION MATRICES
  note: REQUIRED LINEAR/ANGULAR VELOCITIES
  note: GEOMETRIC PROPERTIES
  note: Form relevant linear/angular velocities per (33) - (34).
  note: LINEAR/ANGULAR VELOCITIES
  note: ROTATION MATRICES
  xt2 : Inport
  dxt2r : Inport  Port=2
  WRotXRS2 : Inport  Port=3
  velsRS2 : Inport  Port=4
  velsRS2req : Inport  Port=5
  sbGeomPropPS2 : Subsystem
  sbPosVecsPS2 : Subsystem
  sbRotMatsPS2 : Subsystem
  sbUMatsPS2 : Subsystem
  sbVelsPS2 : Subsystem
  sbVelsPS2req : Subsystem
  geomPropPS2 : Outport
  posVecsPS2 : Outport  Port=2
  WRotXPS2 : Outport  Port=3
  UMatsPS2 : Outport  Port=4
  velsPS2 : Outport  Port=5
  velsPS2req : Outport  Port=6
  wires:
  [velsPS2] -> velsPS2/1  "velsPS2"
  sbVelsPS2/1(velsPS2) -> [velsPS2]  "velsPS2"
  [UMatsPS2] -> sbVelsPS2/2(UMatsPS2)  "UMatsPS2"
  [geomPropPS2] -> sbVelsPS2/1(geomPropPS2)  "geomPropPS2"
  [velsRS2] -> sbVelsPS2/3(velsRS2)  "velsRS2"
  [UMatsPS2] -> UMatsPS2/1  "UMatsPS2"
  sbUMatsPS2/1(UMatsPS2) -> [UMatsPS2]  "UMatsPS2"
  [rotMatsPS2] -> sbUMatsPS2/2(rotMatsPS2)  "rotMatsPS2"
  [posVecsPS2] -> sbUMatsPS2/1(posVecsPS2)  "posVecsPS2"
  sbRotMatsPS2/1(rotMatsPS2) -> [rotMatsPS2]  "rotMatsPS2"
  [WRotXPS2] -> WRotXPS2/1  "WRotXPS2"
  [WRotXRS2] -> sbRotMatsPS2/1(WRotXRS2)  "WRotXRS2"
  sbRotMatsPS2/2(WRotXPS2) -> [WRotXPS2]  "WRotXPS2"
  [posVecsPS2] -> posVecsPS2/1  "posVecsPS2"
  [xt2] -> sbPosVecsPS2/1(xt2)  "xt2"
  sbPosVecsPS2/1(posVecsPS2) -> [posVecsPS2]  "posVecsPS2"
  [xt2] -> sbGeomPropPS2/1(xt2)  "xt2"
  [geomPropPS2] -> geomPropPS2/1  "geomPropPS2"
  WRotXRS2/1 -> [WRotXRS2]  "WRotXRS2"
  velsRS2/1 -> [velsRS2]  "velsRS2"
  xt2/1 -> [xt2]  "xt2"
  dxt2r/1 -> [dxt2r]  "dxt2r"
  velsRS2req/1 -> [velsRS2req]  "velsRS2req"
  [velsPS2req] -> velsPS2req/1  "velsPS2req"
  [velsRS2req] -> sbVelsPS2req/3(velsRS2req)  "velsRS2req"
  [dxt2r] -> sbVelsPS2req/1(dxt2r)  "dxt2r"
  [UMatsPS2] -> sbVelsPS2req/2(UMatsPS2)  "UMatsPS2"
  sbVelsPS2req/1(velsPS2req) -> [velsPS2req]  "velsPS2req"
  sbGeomPropPS2/1(geomPropPS2) -> [geomPropPS2]  "geomPropPS2"

== system VDCHyd2022a/sbVDCController/sbFormAnalyticQuantities/sbRevoluteSegment1 ==
  note: Form relevant linear/angular velocities per (25) - (31).
  note: Form relevant velocity/force transformation matrices...
  note: Form relevant rotation matrices...
  note: Form relevant position vectors...
  note: Get inputs...
  note: Calculate kinematic quantities (18) - (23) in the revolute segment 1 (RS1).
  note: Process data...
  note: Pass to outputs...
  note: Form relevant linear/angular velocities per (39) - (45).
  note: Re-calculate kinematic quantities (21) - (23) in the revolute segment 1 (RS1) using required joint angle.
  note: GEOMETRIC PROPERTIES
  note: REQUIRED GEOMETRIC PROPERTIES
  note: POSITION VECTORS
  note: ROTATION MATRICES
  note: VELOCITY/FORCE TRANSFORMATION MATRICES
  note: LINEAR/ANGULAR VELOCITIES
  note: REQUIRED LINEAR/ANGULAR VELOCITIES
  q1 : Inport  Unit=rad
  dq1r : Inport  Port=2  Unit=rad/s
  WRotBc1 : Inport  Port=3
  Bc1_V : Inport  Port=4  PortDimensions=[6 1]
  Bc1_Vr : Inport  Port=5  Unit=rad
  sbGeomPropRS1 : Subsystem
  sbGeomPropRS1req : Subsystem
  sbPosVecsRS1 : Subsystem
  sbRotMatsRS1 : Subsystem
  sbUMatsRS1 : Subsystem
  sbVelsRS1 : Subsystem
  sbVelsRS1req : Subsystem
  geomPropRS1 : Outport
  geomPropRS1req : Outport  Port=2
  posVecsRS1 : Outport  Port=3
  WRotXRS1 : Outport  Port=4
  UMatsRS1 : Outport  Port=5
  velsRS1 : Outport  Port=6
  velsRS1req : Outport  Port=7
  wires:
  [posVecsRS1] -> posVecsRS1/1  "posVecsRS1"
  [q1] -> sbGeomPropRS1/1(q1)  "q1"
  q1/1 -> [q1]  "q1"
  [WRotXRS1] -> WRotXRS1/1  "WRotXRS1"
  sbRotMatsRS1/2(WRotXRS1) -> [WRotXRS1]  "WRotXRS1"
  [UMatsRS1] -> UMatsRS1/1  "UMatsRS1"
  [WRotBc1] -> sbRotMatsRS1/2(WRotBc1)  "WRotBc1"
  WRotBc1/1 -> [WRotBc1]  "WRotBc1"
  [Bc1V] -> sbVelsRS1/3(Bc1_V)  "Bc1V"
  Bc1_V/1 -> [Bc1V]  "Bc1V"
  [UMatsRS1] -> sbVelsRS1/2(UMatsRS1)  "UMatsRS1"
  sbUMatsRS1/1(UMatsRS1) -> [UMatsRS1]  "UMatsRS1"
  [velsRS1] -> velsRS1/1  "velsRS1"
  sbVelsRS1/1(velsRS1) -> [velsRS1]  "velsRS1"
  [geomPropRS1] -> geomPropRS1/1  "geomPropRS1"
  [posVecsRS1] -> sbUMatsRS1/1(posVecsRS1)  "posVecsRS1"
  sbPosVecsRS1/1(posVecsRS1) -> [posVecsRS1]  "posVecsRS1"
  [rotMatsRS1] -> sbUMatsRS1/2(rotMatsRS1)  "rotMatsRS1"
  sbRotMatsRS1/1(rotMatsRS1) -> [rotMatsRS1]  "rotMatsRS1"
  [geomPropRS1] -> sbVelsRS1/1(geomPropRS1)  "geomPropRS1"
  [geomPropRS1] -> sbRotMatsRS1/1(geomPropRS1)  "geomPropRS1"
  [geomPropRS1] -> sbPosVecsRS1/1(geomPropRS1)  "geomPropRS1"
  sbGeomPropRS1/1(geomPropRS1) -> [geomPropRS1]  "geomPropRS1"
  sbVelsRS1req/1(velsRS1req) -> [velsRS1req]  "velsRS1req"
  [UMatsRS1] -> sbVelsRS1req/2(UMatsRS1)  "UMatsRS1"
  [Bc1Vr] -> sbVelsRS1req/3(Bc1Vr)  "Bc1Vr"
  sbGeomPropRS1req/1(geomPropRS1req) -> [geomPropRS1req]  "geomPropRS1req"
  [dq1r] -> sbGeomPropRS1req/2(dq1r)  "dq1r"
  [geomPropRS1req] -> sbVelsRS1req/1(geomPropRS1req)  "geomPropRS1req"
  [velsRS1req] -> velsRS1req/1  "velsRS1req"
  [geomPropRS1] -> sbGeomPropRS1req/1(geomPropRS1)  "geomPropRS1"
  dq1r/1 -> [dq1r]  "dq1r"
  Bc1_Vr/1 -> [Bc1Vr]  "Bc1_Vr"
  [geomPropRS1req] -> geomPropRS1req/1  "geomPropRS1req"

== system VDCHyd2022a/sbVDCController/sbFormAnalyticQuantities/sbRevoluteSegment2 ==
  note: Due to repeatable nature of the calculation process, all the comments in RS1 remain generally the same in RS2.
  note: Get inputs...
  note: Process data...
  note: Pass to outputs...
  note: POSITION VECTORS
  note: REQUIRED GEOMETRIC PROPERTIES
  note: VELOCITY/FORCE TRANSFORMATION MATRICES
  note: REQUIRED LINEAR/ANGULAR VELOCITIES
  note: GEOMETRIC PROPERTIES
  note: LINEAR/ANGULAR VELOCITIES
  note: ROTATION MATRICES
  note: Re-calculate kinematic quantities (21) - (23) in the revolute segment 2 (RS2) using required joint angle.
  note: Calculate kinematic quantities (18) - (23) in the revolute segment 2 (RS2).
  note: Form relevant rotation matrices...
  note: Form relevant position vectors...
  note: Form relevant linear/angular velocities per (39) - (45).
  note: Form relevant linear/angular velocities per (25) - (31).
  note: Form relevant velocity/force transformation matrices...
  q2 : Inport
  dq2r : Inport  Port=2
  WRotXRS1 : Inport  Port=3
  velsRS1 : Inport  Port=4
  velsRS1req : Inport  Port=5
  sbGeomPropRS2 : Subsystem
  sbGeomPropRS2req : Subsystem
  sbPosVecsRS2 : Subsystem
  sbRotMatsRS2 : Subsystem
  sbUMatsRS2 : Subsystem
  sbVelsRS2 : Subsystem
  sbVelsRS2req : Subsystem
  geomPropRS2 : Outport
  geomPropRS2req : Outport  Port=2
  posVecsRS2 : Outport  Port=3
  WRotXRS2 : Outport  Port=4
  UMatsRS2 : Outport  Port=5
  velsRS2 : Outport  Port=6
  velsRS2req : Outport  Port=7
  wires:
  [velsRS2] -> velsRS2/1  "velsRS2"
  sbVelsRS2/1(velsRS2) -> [velsRS2]  "velsRS2"
  [WRotXRS1] -> sbRotMatsRS2/2(WRotXRS1)  "WRotXRS1"
  WRotXRS1/1 -> [WRotXRS1]  "WRotXRS1"
  [velsRS1] -> sbVelsRS2/3(velsRS1)  "velsRS1"
  velsRS1/1 -> [velsRS1]  "velsRS1"
  [WRotXRS2] -> WRotXRS2/1  "WRotXRS2"
  sbRotMatsRS2/2(WRotXRS2) -> [WRotXRS2]  "WRotXRS2"
  [UMatsRS2] -> UMatsRS2/1  "UMatsRS2"
  [UMatsRS2] -> sbVelsRS2/2(UMatsRS2)  "UMatsRS2"
  sbUMatsRS2/1(UMatsRS2) -> [UMatsRS2]  "UMatsRS2"
  [rotMatsRS2] -> sbUMatsRS2/2(rotMatsRS2)  "rotMatsRS2"
  [posVecsRS2] -> posVecsRS2/1  "posVecsRS2"
  [posVecsRS2] -> sbUMatsRS2/1(posVecsRS2)  "posVecsRS2"
  sbPosVecsRS2/1(posVecsRS2) -> [posVecsRS2]  "posVecsRS2"
  q2/1 -> [q2]  "q2"
  sbRotMatsRS2/1(rotMatsRS2) -> [rotMatsRS2]  "rotMatsRS2"
  [geomPropRS2] -> geomPropRS2/1  "geomPropRS2"
  [q2] -> sbGeomPropRS2/1(q2)  "q2"
  sbGeomPropRS2/1(geomPropRS2) -> [geomPropRS2]  "geomPropRS2"
  [geomPropRS2] -> sbPosVecsRS2/1(geomPropRS2)  "geomPropRS2"
  [geomPropRS2] -> sbRotMatsRS2/1(geomPropRS2)  "geomPropRS2"
  [geomPropRS2] -> sbVelsRS2/1(geomPropRS2)  "geomPropRS2"
  [velsRS2req] -> velsRS2req/1  "velsRS2req"
  sbGeomPropRS2req/1(geomPropRS2req) -> [geomPropRS2req]  "geomPropRS2req"
  [dq2r] -> sbGeomPropRS2req/2(dq2r)  "dq2r"
  [geomPropRS2] -> sbGeomPropRS2req/1(geomPropRS2)  "geomPropRS2"
  [geomPropRS2req] -> sbVelsRS2req/1(geomPropRS2req)  "geomPropRS2req"
  [UMatsRS2] -> sbVelsRS2req/2(UMatsRS2)  "UMatsRS2"
  [velsRS1req] -> sbVelsRS2req/3(velsRS1req)  "velsRS1req"
  sbVelsRS2req/1(velsRS2req) -> [velsRS2req]  "velsRS2req"
  dq2r/1 -> [dq2r]  "dq2r"
  velsRS1req/1 -> [velsRS1req]  "velsRS1req"
  [geomPropRS2req] -> geomPropRS2req/1  "geomPropRS2req"

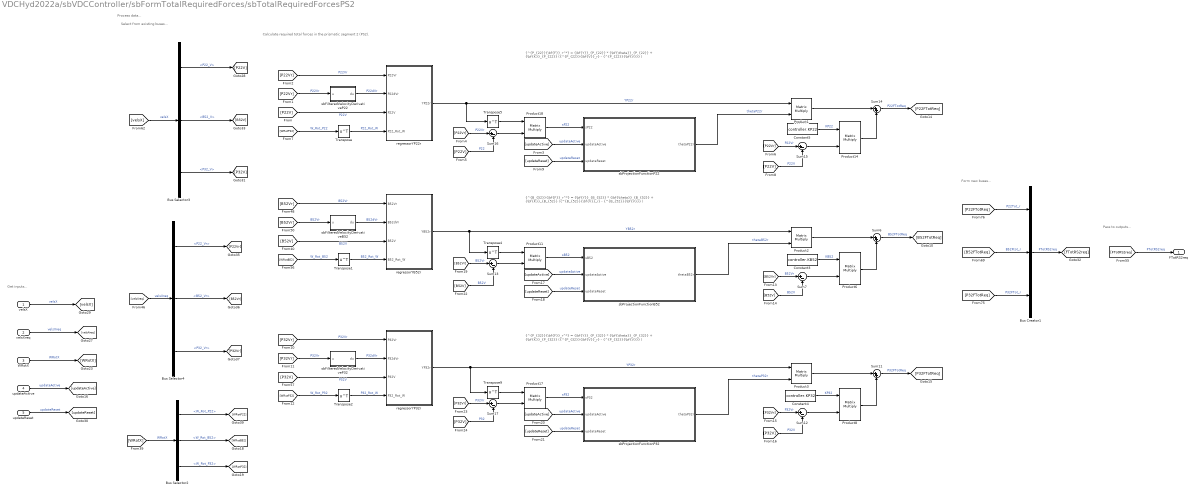
== system VDCHyd2022a/sbVDCController/sbFormTotalRequiredForces/sbTotalRequiredForcesPS2 ==
  note: Form new buses...
  note: Pass to outputs...
  note: Process data...
  note: Get inputs...
  note: Select from existing buses...
  note: Calculate required total forces in the prismatic segment 2 (PS2).
  note: {^{P_{22}}{\bf{F}}_r^*} = {\bf{Y}}_{P_{22}} * {\bf{\theta}}_{P_{22}} + {\bf{K}}_{P_{22}} ({^{P_{22}}{\bf{V}}_r} - {^{P_{22}}{\bf{V}}} )
  note: {^{B_{52}}{\bf{F}}_r^*} = {\bf{Y}}_{B_{52}} * {\bf{\theta}}_{B_{52}} + {\bf{K}}_{B_{52}} ({^{B_{52}}{\bf{V}}_r} - {^{B_{52}}{\bf{V}}} )
  note: {^{P_{32}}{\bf{F}}_r^*} = {\bf{Y}}_{P_{32}} * {\bf{\theta}}_{P_{32}} + {\bf{K}}_{P_{32}} ({^{P_{32}}{\bf{V}}_r} - {^{P_{32}}{\bf{V}}} )
  velsX : Inport
  velsXreq : Inport  Port=2
  WRotX : Inport  Port=3
  updateActive : Inport  Port=4
  updateReset : Inport  Port=5
  Bus Creator1 : BusCreator  Inputs=P22Tot_r,B52Ftot_r,P32FTot_r
  Bus Selector2 : BusSelector  OutputSignals=WRotXRS2.W_Rot_P22,WRotXPS2.W_Rot_B52,WRotXPS2.W_Rot_P32
  Bus Selector3 : BusSelector  OutputSignals=velsRS2.P22_V,velsPS2.B52_V,velsPS2.P32_V
  Bus Selector4 : BusSelector  OutputSignals=velsRS2req.P22_Vr,velsPS2req.B52_Vr,velsPS2req.P32_Vr
  Constant3 : Constant  Value=controller.KB52
  Constant4 : Constant  Value=controller.KP32
  Constant5 : Constant  Value=controller.KP22
  Product{1..3,6,8,11,14,17..18} (9 alike) : Product  Multiplication=Matrix(*)
  Sum11 : Sum  Inputs=|++
  Sum{7,12..13,15..17} (6 alike) : Sum  Inputs=|+-
  Sum14 : Sum  Inputs=|++
  Sum6 : Sum  Inputs=|++
  Transpose{,1..2,4..5,9} (6 alike) : Math  Operator=transpose
  regressorYB52r : MATLAB Function  TreatAsAtomicUnit=on
  regressorYP22r : MATLAB Function  TreatAsAtomicUnit=on
  regressorYP32r : MATLAB Function  TreatAsAtomicUnit=on
  sbFilteredVelocityDerivativeB52 : Subsystem
  sbFilteredVelocityDerivativeP22 : Subsystem
  sbFilteredVelocityDerivativeP32 : Subsystem
  sbProjectionFunctionB52 : Subsystem
  sbProjectionFunctionP22 : Subsystem
  sbProjectionFunctionP32 : Subsystem
  FTotRS2req : Outport
  wires:
  velsXreq/1 -> [velsXreq]  "velsXreq"
  [B52FTotReq] -> Bus Creator1/2  "B52Ftot_r"
  Bus Selector3/3 -> [P32V]  "<P32_V>"
  Bus Selector4/3 -> [P32Vr]  "<P32_Vr>"
  velsX/1 -> [velsX]  "velsX"
  Bus Selector4/2 -> [B52Vr]  "<B52_Vr>"
  Bus Selector3/2 -> [B52V]  "<B52_V>"
  Bus Selector4/1 -> [P22Vr]  "<P22_Vr>"
  [velsXreq] -> Bus Selector4/1  "velsXreq"
  Bus Selector2/3 -> [WRotP32]  "<W_Rot_P32>"
  updateActive/1 -> [updateActive]  "updateActive"
  WRotX/1 -> [WRotX]  "WRotX"
  [velsX] -> Bus Selector3/1  "velsX"
  Bus Selector2/2 -> [WRotB52]  "<W_Rot_B52>"
  [FTotRS2req] -> FTotRS2req/1  "FTotRS2req"
  [P32FTotReq] -> Bus Creator1/3  "P32FTot_r"
  [P22FTotReq] -> Bus Creator1/1  "P22Tot_r"
  updateReset/1 -> [updateReset]  "updateReset"
  [WRotX] -> Bus Selector2/1  "WRotX"
  Bus Selector2/1 -> [WRotP22]  "<W_Rot_P22>"
  Bus Selector3/1 -> [P22V]  "<P22_V>"
  Bus Creator1/1 -> [FTotRS2req]  "FTotRS2req"
  Product2/1 -> Sum6/1
  [P32V] -> regressorYP32r/3(P32V)  "P32V"
  Constant3/1 -> Product6/1  "KB52"
  [B52Vr] -> Sum7/1  "B52Vr"
  [P32Vr] -> Sum17/1  "P32Vr"
  [WRotP32] -> Transpose2/1  "W_Rot_P32"
  [P22V] -> Sum16/2  "P22"
  Product8/1 -> Sum11/2
  Transpose5/1 -> Product18/1
  [WRotB52] -> Transpose1/1  "W_Rot_B52"
  [P32Vr] -> regressorYP32r/1(P32Vr)  "P32Vr"
  [P22Vr] -> regressorYP22r/1(P22Vr)  "P22Vr"
  [P22Vr] -> Sum15/1  "P22Vr"
  Product17/1 -> sbProjectionFunctionP32/1(sP32)  "sP32"
  regressorYP32r/1(YP32r) -> Product3/1, Transpose9/1  "YP32r"
  sbProjectionFunctionB52/1(thetaB52r) -> Product2/2  "thetaB52r"
  regressorYB52r/1(YB52r) -> Product2/1, Transpose4/1  "YB52r"
  [WRotP22] -> Transpose/1  "W_Rot_P22"
  [B52V] -> regressorYB52r/3(B52V)  "B52V"
  [P32Vr] -> sbFilteredVelocityDerivativeP32/1(u)  "P32Vr"
  Transpose1/1 -> regressorYB52r/4(B52_Rot_W)  "B52_Rot_W"
  [P22V] -> Sum15/2  "P22V"
  [P22V] -> regressorYP22r/3(P22V)  "P22V"
  Transpose2/1 -> regressorYP32r/4(P32_Rot_W)  "P32_Rot_W"
  [P32V] -> Sum12/2  "P32V"
  sbFilteredVelocityDerivativeP22/1(du) -> regressorYP22r/2(P22dVr)  "P22dVr"
  [B52V] -> Sum7/2  "B52V"
  Transpose4/1 -> Product11/1
  Constant4/1 -> Product8/1  "KP32"
  Sum12/1 -> Product8/2
  Sum14/1 -> [P22FTotReq]  "P22FTotReq"
  Sum15/1 -> Product14/2
  Constant5/1 -> Product14/1  "KP22"
  [P32Vr] -> Sum12/1  "P32Vr"
  Product6/1 -> Sum6/2
  [B52Vr] -> regressorYB52r/1(B52Vr)  "B52Vr"
  Product1/1 -> Sum14/1
  Sum11/1 -> [P32FTotReq]  "P32FTotReq"
  Sum6/1 -> [B52FTotReq]  "B52FTotReq"
  Sum7/1 -> Product6/2
  sbFilteredVelocityDerivativeB52/1(du) -> regressorYB52r/2(B52dVr)  "B52dVr"
  [B52Vr] -> sbFilteredVelocityDerivativeB52/1(u)  "B52Vr"
  sbFilteredVelocityDerivativeP32/1(du) -> regressorYP32r/2(P32dVr)  "P32dVr"
  Product3/1 -> Sum11/1
  Product14/1 -> Sum14/2
  [B52Vr] -> Sum13/1  "B52Vr"
  [P32V] -> Sum17/2  "P32"
  Product18/1 -> sbProjectionFunctionP22/1(sP22)  "sP22"
  Product11/1 -> sbProjectionFunctionB52/1(sB52)  "sB52"
  Transpose/1 -> regressorYP22r/4(P22_Rot_W)  "P22_Rot_W"
  [P22Vr] -> sbFilteredVelocityDerivativeP22/1(u)  "P22Vr"
  Transpose9/1 -> Product17/1
  Sum16/1 -> Product18/2
  [B52V] -> Sum13/2  "B52V"
  sbProjectionFunctionP32/1(thetaP32r) -> Product3/2  "thetaP32r"
  [P22Vr] -> Sum16/1  "P22Vr"
  regressorYP22r/1(YP22r) -> Product1/1, Transpose5/1  "YP22r"
  sbProjectionFunctionP22/1(thetaP22r) -> Product1/2  "thetaP22r"
  Sum13/1 -> Product11/2
  Sum17/1 -> Product17/2
  [updateActive] -> sbProjectionFunctionP22/2(updateActive)  "updateActive"
  [updateReset] -> sbProjectionFunctionP22/3(updateReset)  "updateReset"
  [updateReset] -> sbProjectionFunctionB52/3(updateReset)  "updateReset"
  [updateActive] -> sbProjectionFunctionB52/2(updateActive)  "updateActive"
  [updateReset] -> sbProjectionFunctionP32/3(updateReset)  "updateReset"
  [updateActive] -> sbProjectionFunctionP32/2(updateActive)  "updateActive"
